simulink model "Simulink_PID"  (Simulink 10.3)
settings: Solver=ode45  StartTime=0.0  StopTime=5e-3  RelTol=1e-3  EnableMultiTasking=on
undefined symbols (not defined in the file or in its folder): den_la, num_la
libraries: simulink x3
settings Model: Creator=alumno  LastModifiedBy=franf
settings DataIOCC: LimitDataPoints=on
settings SFSimCC: SimUserSources=C:\MATLAB2012aPortable  SimUserIncludeDirs=C:\MATLAB2012aPortable  SimUserLibraries=C:\MATLAB2012aPortable
settings GRTTargetCC: CombineOutputUpdateFcns=on  GRTInterface=off

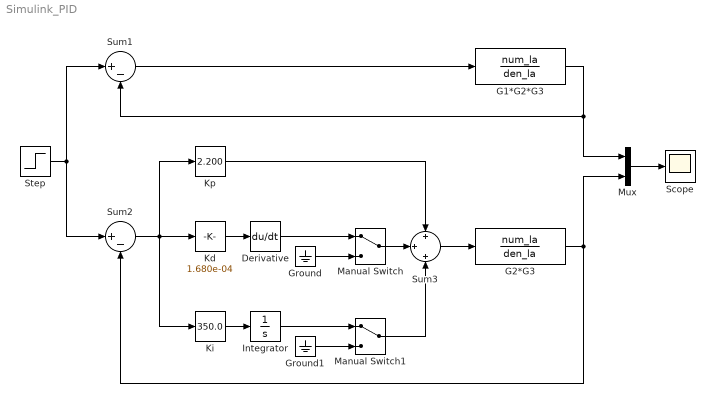
== system Simulink_PID ==
  Derivative : Derivative
  G1*G2*G3 : TransferFcn  Numerator=num_la  Denominator=den_la
  G2*G3 : TransferFcn  Numerator=num_la  Denominator=den_la
  Ground : Ground
  Ground1 : Ground
  Integrator : Integrator
  Kd : simulink/Math Operations/Slider Gain  gain=1.680e-04  low=0  high=0.0006
  Ki : simulink/Math Operations/Slider Gain  gain=350.0  low=0  high=5000
  Kp : simulink/Math Operations/Slider Gain  gain=2.200  low=0  high=10
  Manual Switch : ManualSwitch
  Manual Switch1 : ManualSwitch
  Mux : Mux  Inputs=2
  Scope : Scope
  Step : Step  Time=0  SampleTime=0
  Sum1 : Sum  Inputs=|+-
  Sum2 : Sum  Inputs=|+-
  Sum3 : Sum  Inputs=+|+|+
  wires:
  Kd/1 -> Derivative/1
  Ki/1 -> Integrator/1
  Kp/1 -> Sum3/1
  Sum2/1 -> Ki/1, Kp/1, Kd/1
  Sum3/1 -> G2*G3/1
  Manual Switch/1 -> Sum3/2
  Derivative/1 -> Manual Switch/1
  Ground/1 -> Manual Switch/2
  Manual Switch1/1 -> Sum3/3
  Integrator/1 -> Manual Switch1/1
  Ground1/1 -> Manual Switch1/2
  G2*G3/1 -> Mux/2, Sum2/2
  Sum1/1 -> G1*G2*G3/1
  Step/1 -> Sum2/1, Sum1/1
  G1*G2*G3/1 -> Mux/1, Sum1/2
  Mux/1 -> Scope/1
